simulink model "balancing_flow"  (R2023a)
settings: Solver=VariableStepAuto  StartTime=0.0  StopTime=10.0  RelTol=1e-3
InitFcn:
  | %% start clustering
  | %clear;
  | load('workspace.mat');
  | cell_count = 9;
  | soc = fix(rand (1, cell_count) * 100);
  | mp  = 2;
  | ep = 10;
  | [cluster] = pso_DBSCAN(soc, mp, ep);
values from neighbouring files (symbols this model uses):
  cluster =     [workspace.mat]
settings Model: Creator=Mahdi  LastModifiedBy=Mahdi

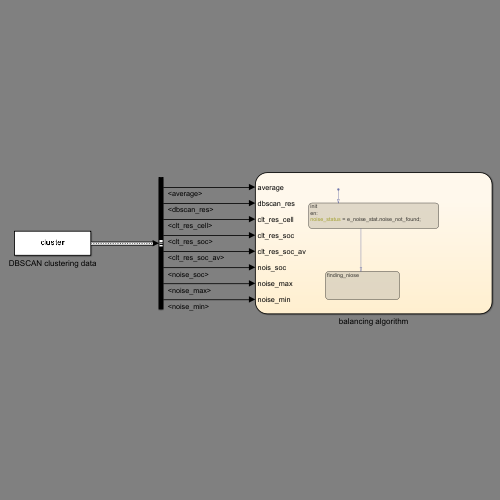
[thumbnail: Simulink's stored preview of the top-level diagram]
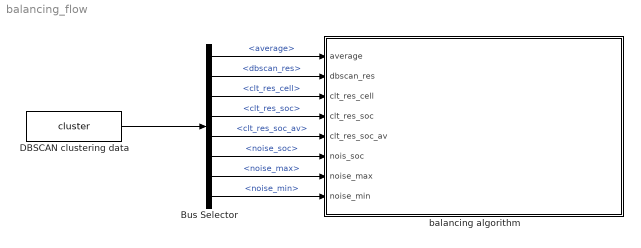
== system balancing_flow ==
  Bus Selector : BusSelector  OutputSignals=average,dbscan_res,clt_res_cell,clt_res_soc,clt_res_soc_av,noise_soc,noise_max,noise_min
  DBSCAN clustering data : Constant  Value=cluster  OutDataTypeStr=Bus: cluster_bus
  balancing algorithm : Stateflow chart  TreatAsAtomicUnit=on
  wires:
  DBSCAN clustering data/1 -> Bus Selector/1
  Bus Selector/1 -> balancing algorithm/1(average)  "<average>"
  Bus Selector/2 -> balancing algorithm/2(dbscan_res)  "<dbscan_res>"
  Bus Selector/3 -> balancing algorithm/3(clt_res_cell)  "<clt_res_cell>"
  Bus Selector/4 -> balancing algorithm/4(clt_res_soc)  "<clt_res_soc>"
  Bus Selector/5 -> balancing algorithm/5(clt_res_soc_av)  "<clt_res_soc_av>"
  Bus Selector/6 -> balancing algorithm/6(nois_soc)  "<noise_soc>"
  Bus Selector/7 -> balancing algorithm/7(noise_max)  "<noise_max>"
  Bus Selector/8 -> balancing algorithm/8(noise_min)  "<noise_min>"

== stateflow chart balancing_flow/balancing algorithm ==
  state init
    en:
    noise_status = e_noise_stat.noise_not_found;
  state finding_niose
  (default) -> init
  init -> finding_niose
  data: noise_status local; average input; dbscan_res input; clt_res_cell input; clt_res_soc input; clt_res_soc_av input; nois_soc input; noise_max input; noise_min input
